simulink model "sim_MPC_Heli_integral"  (R2020a)
settings: Solver=ode4  StartTime=0.0  StopTime=inf  FixedStep=0.01  RelTol=1e-3
InitFcn:
  | run('initialize_system.m')
values from neighbouring files (symbols this model uses):
  Ac = At    [initialize_system_du.m]
  Ad = ds.a    [initialize_system.m]    (also in initialize_system_du.m)
  Bc = Bt    [initialize_system_du.m]
  Bd = ds.b    [initialize_system.m]    (also in initialize_system_du.m)
  Cc = Ct    [initialize_system_du.m]
  Cd = ds.c    [initialize_system.m]    (also in initialize_system_du.m)
  th_op = -10*pi/180    (= -0.174532925199)    [initialize_system.m]    (also in initialize_system_du.m)
  Vmp_op = (Kyy*m_heli*g*cos(th_op)*l_cm) / (Kyy*Kpp - Kyp*Kpy)    [initialize_system.m]    (also in initialize_system_du.m)
  Vmy_op = (Kyp*Vmp_op) / (Kyy)    [initialize_system.m]    (also in initialize_system_du.m)
  w_th_op = 0    [initialize_system.m]    (also in initialize_system_du.m)
  w_yw_op = 0    [initialize_system.m]    (also in initialize_system_du.m)
  yw_op = pi/2    (= 1.57079632679)    [initialize_system.m]    (also in initialize_system_du.m)
undefined symbols (not defined in the file or in its folder): L
libraries: simulink_extras x3, realtime_pacer_lib x1
(part 2 of 2)

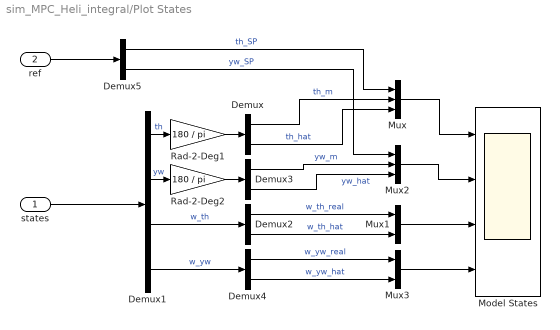
== system sim_MPC_Heli_integral/Plot States ==
  states : Inport
  ref : Inport  Port=2
  Demux{,2..5} (5 alike) : Demux  Outputs=2
  Demux1 : Demux
  Model States : Scope  NumInputPorts=4
  Mux : Mux  Inputs=3
  Mux1 : Mux  Inputs=2
  Mux2 : Mux  Inputs=3
  Mux3 : Mux  Inputs=2
  Rad-2-Deg1 : Gain  Gain=180 / pi
  Rad-2-Deg2 : Gain  Gain=180 / pi
  wires:
  states/1 -> Demux1/1
  Demux/1 -> Mux/2  "th_m"
  Demux/2 -> Mux/3  "th_hat"
  Demux3/1 -> Mux2/2  "yw_m"
  Demux3/2 -> Mux2/3  "yw_hat"
  Demux2/1 -> Mux1/1  "w_th_real"
  Demux2/2 -> Mux1/2  "w_th_hat"
  Demux4/1 -> Mux3/1  "w_yw_real"
  Demux4/2 -> Mux3/2  "w_yw_hat"
  Demux1/1 -> Rad-2-Deg1/1  "th"
  Demux1/2 -> Rad-2-Deg2/1  "yw"
  Demux1/3 -> Demux2/1  "w_th"
  Demux1/4 -> Demux4/1  "w_yw"
  Mux/1 -> Model States/1
  Mux2/1 -> Model States/2
  Mux1/1 -> Model States/3
  Mux3/1 -> Model States/4
  ref/1 -> Demux5/1
  Demux5/2 -> Mux2/1  "yw_SP"
  Demux5/1 -> Mux/1  "th_SP"
  Rad-2-Deg1/1 -> Demux/1
  Rad-2-Deg2/1 -> Demux3/1

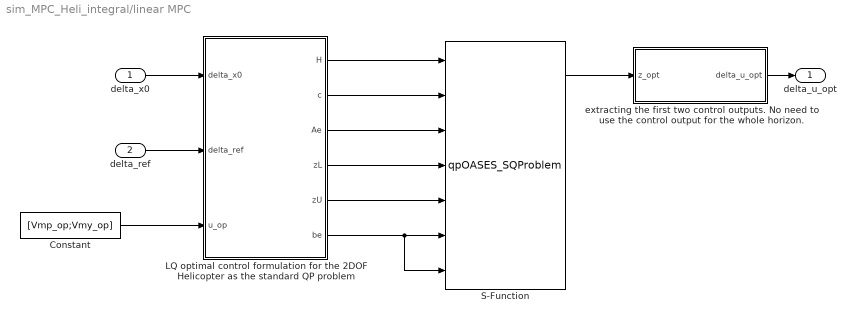
== system sim_MPC_Heli_integral/linear MPC ==
  delta_x0 : Inport
  delta_ref : Inport  Port=2
  Constant : Constant  Value=[Vmp_op;Vmy_op]
  LQ optimal control formulation for the 2DOF Helicopter as the standard QP problem : MATLAB Function  TreatAsAtomicUnit=on
  S-Function : S-Function  FunctionName=qpOASES_SQProblem  SFunctionDeploymentMode=off  EnableBusSupport=off
  extracting the first two control outputs. No need to use the control output for the whole horizon. : MATLAB Function  TreatAsAtomicUnit=on
  delta_u_opt : Outport
  wires:
  delta_x0/1 -> LQ optimal control formulation for the 2DOF Helicopter as the standard QP problem/1(delta_x0)
  delta_ref/1 -> LQ optimal control formulation for the 2DOF Helicopter as the standard QP problem/2(delta_ref)
  LQ optimal control formulation for the 2DOF Helicopter as the standard QP problem/1(H) -> S-Function/1
  LQ optimal control formulation for the 2DOF Helicopter as the standard QP problem/2(c) -> S-Function/2
  LQ optimal control formulation for the 2DOF Helicopter as the standard QP problem/3(Ae) -> S-Function/3
  LQ optimal control formulation for the 2DOF Helicopter as the standard QP problem/4(zL) -> S-Function/4
  LQ optimal control formulation for the 2DOF Helicopter as the standard QP problem/5(zU) -> S-Function/5
  LQ optimal control formulation for the 2DOF Helicopter as the standard QP problem/6(be) -> S-Function/7, S-Function/6
  S-Function/1 -> extracting the first two control outputs. No need to use the control output for the whole horizon./1(z_opt)
  extracting the first two control outputs. No need to use the control output for the whole horizon./1(delta_u_opt) -> delta_u_opt/1
  Constant/1 -> LQ optimal control formulation for the 2DOF Helicopter as the standard QP problem/3(u_op)

== matlab function sim_MPC_Heli_integral/Linear State Observer/Kalman Filter ==
  data: delta_x input; delta_u input; delta_x_hat output size=4; delta_y_m input; Ac parameter; Bc parameter; Cc parameter; L parameter
function delta_x_hat = linear_state_observer(delta_x, delta_u,delta_y_m,Ac,Bc,Cc,L)
    %apriori state
    delta_x_hat = Ac*delta_x + Bc*delta_u;
    %estimated output    
    y_hat = Cc*delta_x;
    % aposteriori state
    delta_x_hat = delta_x_hat + L*(delta_y_m - y_hat);

== matlab function sim_MPC_Heli_integral/nonlinear_model ==
  data: Vmp input; d_th_dt output; Vmy input; th input; yw input; w_th input; w_yw input; d_yw_dt output; d_w_th_dt output; d_w_yw_dt output
% Simulink nonlinear model of USN helicopter
% Author: Eirik Engen
% Date: 2020-09-02

function [d_th_dt, d_yw_dt, d_w_th_dt, d_w_yw_dt] = non_linear_model(Vmp, Vmy, th, yw, w_th, w_yw)          %#ok<INUSL>
% function inputs
% Vmp : Model input - Voltage input to Pitch motor/rotor [V]
% Vmy : Model input - Voltage input to Yaw motor/rotor [V]
% th  : Model state - Pitch angle, theta [radians]
% yw  : Model state - Yaw angle, psi [radians]
% w_th: Model state - Pitch angular velocity, omega_theta [radians / s]
% w_yw: Model state - Yaw angular velocity, omega_psi [radians / s]

% System parameters
l_cm   = 0.015;   % [m] - Distance between the pivot point and the center of mass of the helicopter.
m_heli = 0.479;   % [kg] - Total moving mass of the helicopter
J_eq_p = 0.0172;  % [kg-m^2] - Moment of inertia about pitch axis
J_eq_y = 0.0210;  % [kg-m^2] - Moment of inertia about yaw axis
g      = 9.81;    % [m/s^2] - Acceleration due to gravity on planet earth

Kpp    = 0.0556;  % [Nm/V] - Torque constant on pitch axis from pitch motor
Kyy    = 0.21084; % [Nm/V] - Torque constant on yaw axis from yaw motor
Kpy    = 0.005;   % [Nm/V] - Torque constant on pitch axis from yaw motor
Kyp    = 0.15;    % [Nm/V] - Torque constant on yaw axis from pitch motor
Bp     = 0.01;    % [N/V]  - Damping friction factor about pitch axis
By     = 0.08;    % [N/V]  - Damping friction factor about yaw axis

% Differential equations
d_th_dt = w_th;
d_yw_dt = w_yw;
d_w_th_dt = (Kpp*Vmp - ...
    Kpy*Vmy - ...
    Bp*w_th - ...
    m_heli*l_cm^2*w_yw^2*sin(th)*cos(th) - ...
    m_heli*g*l_cm*cos(th)) / ...
    (J_eq_p+m_heli*l_cm^2);
d_w_yw_dt = (Kyp*Vmp - ...
    Kyy*Vmy - ...
    By*w_yw + ...
    2*m_heli*l_cm^2*w_th*w_yw*sin(th)*cos(th)) / ...
    (J_eq_y+m_heli*l_cm^2*cos(th)^2);

== matlab function sim_MPC_Heli_integral/linear MPC/LQ optimal control formulation for the 2DOF Helicopter as the standard QP problem ==
  data: delta_x0 input; H output; delta_ref input; u_op input; c output; Ae output; zL output; zU output; be output; Ad parameter; Bd parameter; Cd parameter
function [H,c,Ae,zL,zU,be] = QP_formulation_Heli(delta_x0,delta_ref, u_op, Ad, Bd, Cd)
    % System matrices of discrete time model is pre-loaded in Simulink and 
    % Ad, Bd and Cd matrices are configured as parameters in this function.
    %
    % Configuration
    N = 20; % prediction horizon length
    %weighting matrices
    Q=diag([1 1]); %tuning weight for error: there are 2 (size(ny))
    P=diag([1e-3 1e-3]);            %tuning weight for inputs: there are 2 (size(nu))
     %size of state-matrix, output-matrix and input-matrix
    nx = size(Ad,1); nu = size(Bd,2); ny = size(Cd,1);
    %size of the unknow vector z
    nz = N*(nx + nu + 2*ny);
    % Define boundaries
    uL = 0*ones(nu,1) - u_op; 
    uU = 3*ones(nu,1) - u_op;
    %% Litt usikker her om boundaries for tilstander er begrensende?
    %% Mulig at det skal defineres til +- inf.
%     xL = [-45*pi/180;0;-inf;-inf];
%     xU = [45*pi/180;pi;inf;inf];
    xL = -inf*ones(nx,1);
    xU = inf*ones(nx,1);
    eL = -inf*ones(ny,1);
    eU = inf*ones(ny,1);
    yL = -inf*ones(ny,1);
    yU = inf*ones(ny,1);
    
    
    %initial values of the states
    x0 = delta_x0;
    
    % Define reference for the whole prediction/simulation length
    % row # 1: pitch angle
    % row # 2: yaw angle
    r = [ones(1,N).*delta_ref(1);                 
         ones(1,N).*delta_ref(2)];    
    
    % build matrices
    H11 = kron(eye(N),P); 
    H22 = zeros(N*nx,N*nx); 
    H33 = kron(eye(N),Q);
    H44 = zeros(N*ny,N*ny);
    H_mat = blkdiag(H11,H22,H33,H44);
    %reshape to vector form to support qpOASES
    H = H_mat(:);
    c = zeros(nz,1);
    %constraints (from process model)
    % State equation reference
    Ae1u = -kron(eye(N),Bd);
    Ae1x = eye(N*nx)-kron(diag(ones(N-abs(-1),1),-1),Ad); 
    Ae1e = zeros(N*nx,N*ny); % eq 1 is states, hence nx rows, and errors are ny cols.
    Ae1y = zeros(N*nx,N*ny);
    be1 = [Ad*x0;zeros((N-1)*nx,1)];
    %Measurement equation reference
    Ae2u = zeros(N*ny,N*nu); % eq 2 is measurement eq, ny cols, nu inputs
    Ae2x = -kron(eye(N),Cd); 
    Ae2e = zeros(N*ny,N*ny); 
    Ae2y = eye(N*ny);
    be2 = zeros(N*ny,1);
    %Error equation reference
    Ae3u = zeros(N*ny,N*nu); % eq 3 is error, ny lines, and nu inputs
    Ae3x = zeros(N*ny,N*nx); 
    Ae3e = eye(N*ny);
    Ae3y = eye(N*ny);
    % reshape r for be3
    be3 = reshape(r,N*ny,1);
    % Define final Ae matrix
    Ae_mat=[Ae1u Ae1x Ae1e Ae1y 
            Ae2u Ae2x Ae2e Ae2y 
            Ae3u Ae3x Ae3e Ae3y];
    %reshape to vector form to support qpOASES
    Ae = Ae_mat(:);
    % Define final be vector
    be=[be1;be2;be3];
    %bounds
    zL=[kron(ones(N,1),uL)
        kron(ones(N,1),xL)
        kron(ones(N,1),eL)
        kron(ones(N,1),yL)]; 
    
    zU=[kron(ones(N,1),uU)
        kron(ones(N,1),xU)
        kron(ones(N,1),eU)
        kron(ones(N,1),yU)];

== matlab function sim_MPC_Heli_integral/linear MPC/extracting the first two control outputs. No need to use the control output for the whole horizon. ==
  data: z_opt input; delta_u_opt output
function delta_u_opt = extract_first_control(z_opt)

delta_u_opt = z_opt(1:2);
